simulink model "MotorPositionControl"  (R2020a)
settings: Solver=VariableStepAuto  StartTime=0.0  StopTime=2  RelTol=1e-3
undefined symbols (not defined in the file or in its folder): Kd, Ki, Kp
settings Model: DataDictionary=DataDictionaryMotorPositionControlPID.sldd  Creator=DELL  LastModifiedBy=DELL

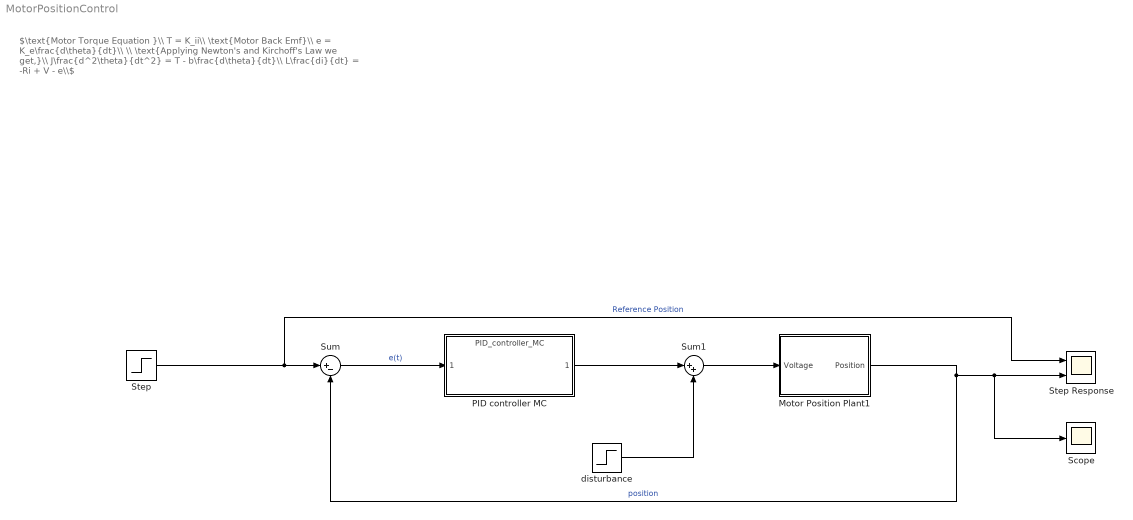
== system MotorPositionControl ==
  note: $\text{Motor Torque Equation }\\ T = K_ii\\ \text{Motor Back Emf}\\ e = K_e\frac{d\theta}{dt}\\ \\ \text{Applying Newton's and Kirchoff's Law we get,}\\ J\frac{d^2\theta}{dt^2} = T - b\frac{d\theta}{dt}\\ L\frac{di}{dt} = -Ri + V - e\\$
  Motor Position Plant1 : Subsystem  mask{J=3.228e-4, b=3.5077e-6, Ke=0.0274, Kt=0.0274, R=4, L=2.75e-6}
      mask prompts: J "Moment of Inertia of the Rotor  [J]"; b "Motor Viscous Friction Constant [b]"; Ke "Electromotive Force Constant  [Ke]"; Kt "Motor Torque Constant            [Kt]"; R "Electrical Resistance                 [R]"; L "Electric Inductance                   [L]"
      mask DialogControl DescGroupVar Prompt: Motor Position Plant
      mask DialogControl DescTextVar Prompt: Motor parameters required.
  PID controller MC : ModelReference  ModelNameDialog=PID_controller_MC  ParameterArgumentNames=Kd,Ki,Kp  ParameterArgumentValues=Kd,Ki,Kp  UsingDefaultArgumentValue=0,0,0  SimulationMode=Normal  ModelReferenceVersion=1.18  Kd=45  Ki=406514  Kp=8718  SimulationMode=Normal
  Scope : Scope
  Step : Step  Time=0.5  SampleTime=0
  Step Response : Scope  NumInputPorts=2
  Sum : Sum  Inputs=|+-
  Sum1 : Sum  Inputs=|++
  "disturbance " : Step  Time=1.5  SampleTime=0
  wires:
  Step/1 -> Step Response/1, Sum/1  "Reference Position"
  Motor Position Plant1/1("Position ") -> Sum/2, Scope/1, Step Response/2  "position"
  Sum/1 -> PID controller MC/1  "e(t)"
  PID controller MC/1 -> Sum1/1
  Sum1/1 -> Motor Position Plant1/1(Voltage)
  "disturbance "/1 -> Sum1/2

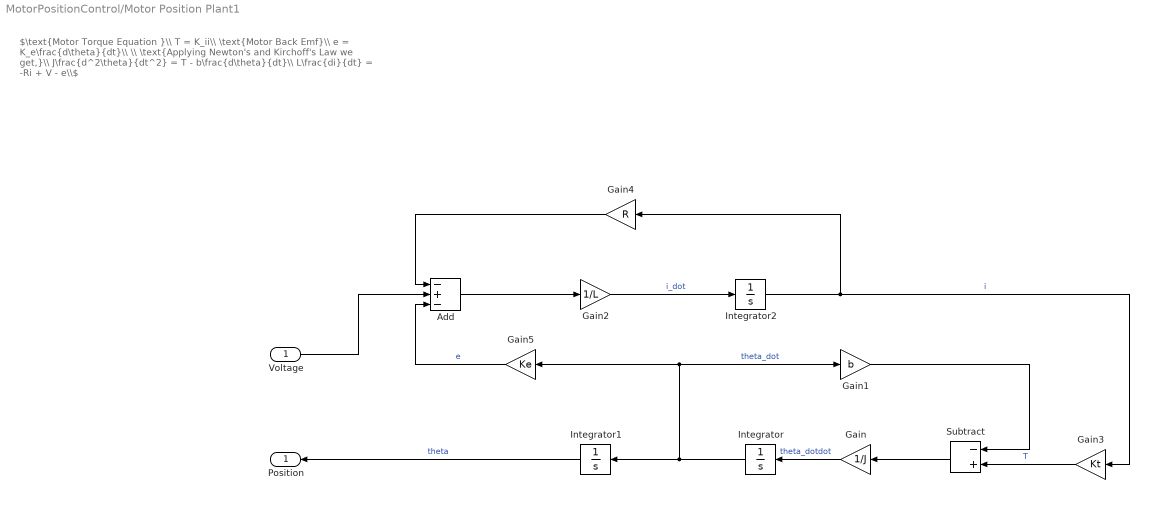
== system MotorPositionControl/Motor Position Plant1 ==
  note: $\text{Motor Torque Equation }\\ T = K_ii\\ \text{Motor Back Emf}\\ e = K_e\frac{d\theta}{dt}\\ \\ \text{Applying Newton's and Kirchoff's Law we get,}\\ J\frac{d^2\theta}{dt^2} = T - b\frac{d\theta}{dt}\\ L\frac{di}{dt} = -Ri + V - e\\$
  Voltage : Inport
  Add : Sum  Inputs=-+-
  Gain : Gain  Gain=1/J
  Gain1 : Gain  Gain=b
  Gain2 : Gain  Gain=1/L
  Gain3 : Gain  Gain=Kt
  Gain4 : Gain  Gain=R
  Gain5 : Gain  Gain=Ke
  Integrator : Integrator
  Integrator1 : Integrator
  Integrator2 : Integrator
  Subtract : Sum  Inputs=-+
  "Position " : Outport
  wires:
  Integrator1/1 -> "Position "/1  "theta"
  Voltage/1 -> Add/2
  Gain/1 -> Integrator/1  "theta_dotdot"
  Integrator2/1 -> Gain3/1, Gain4/1  "i"
  Gain2/1 -> Integrator2/1  "i_dot"
  Gain3/1 -> Subtract/2  "T"
  Gain1/1 -> Subtract/1
  Gain5/1 -> Add/3  "e"
  Subtract/1 -> Gain/1
  Gain4/1 -> Add/1
  Integrator/1 -> Integrator1/1, Gain5/1, Gain1/1  "theta_dot"
  Add/1 -> Gain2/1
